simulink model "bitwise_calc"  (R2021a)
settings: Solver=FixedStepDiscrete  StartTime=0.0  StopTime=10.0  RelTol=1e-3  EnableMultiTasking=on
libraries: simulink x8
settings Model: Creator=Rana  LastModifiedBy=Rana
settings DataIOCC: ReturnWorkspaceOutputs=off
settings OptimizationCC: DefaultParameterBehavior=Inlined  InlineInvariantSignals=on  EnableMemcpy=off  LifeSpan=1  EfficientTunableParamExpr=on
settings DebuggingCC: UnderspecifiedInitializationDetection=Classic  MergeDetectMultiDrivingBlocksExec=none  SFMachineParentedDataDiag=warning  ArithmeticOperatorsInVariantConditions=warning
settings ModelReferenceCC: PropagateSignalLabelsOutOfModel=off
settings SFSimCC: MATLABDynamicMemAlloc=off  CustomCodeUndefinedFunction=UseInterfaceOnly
settings RTWCC: SystemTargetFile=ert.tlc  GenCodeOnly=on  TemplateMakefile=ert_default_tmf  GenerateReport=on  IncludeHyperlinkInReport=on  LaunchReport=on  GenerateTraceInfo=on  GenerateTraceReport=on  GenerateTraceReportSl=on  GenerateTraceReportSf=on  GenerateTraceReportEml=on
settings CodeAppCC: ForceParamTrailComments=on  IgnoreCustomStorageClasses=off  OperatorAnnotations=on  SimulinkDataObjDesc=on  SFDataObjDesc=on  MATLABFcnDesc=on  InsertBlockDesc=on  StateflowObjectComments=on  MATLABSourceComments=on
settings ERTTargetCC: MultiwordLength=2048  GenerateSampleERTMain=on  InlinedParameterPlacement=NonHierarchical  ERTCustomFileTemplate=example_file_process.tlc

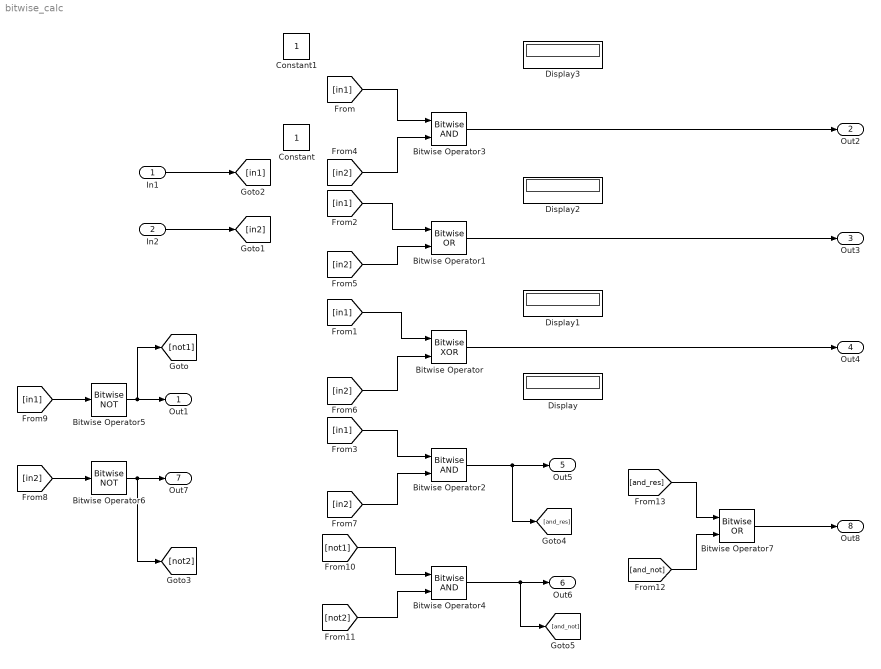
== system bitwise_calc ==
  In1 : Inport  OutDataTypeStr=uint8
  In2 : Inport  Port=2  OutDataTypeStr=uint8
  Bitwise Operator : simulink/Logic and Bit Operations/Bitwise Operator  logicop=XOR  UseBitMask=off  NumInputPorts=2  BitMask=bin2dec('11011001')  BitMaskRealWorld=Stored Integer
  Bitwise Operator1 : simulink/Logic and Bit Operations/Bitwise Operator  logicop=OR  UseBitMask=off  NumInputPorts=2  BitMask=bin2dec('11011001')  BitMaskRealWorld=Stored Integer
  Bitwise Operator2 : simulink/Logic and Bit Operations/Bitwise Operator  logicop=AND  UseBitMask=off  NumInputPorts=2  BitMask=bin2dec('11011001')  BitMaskRealWorld=Stored Integer
  Bitwise Operator3 : simulink/Logic and Bit Operations/Bitwise Operator  logicop=AND  UseBitMask=off  NumInputPorts=2  BitMask=bin2dec('11011001')  BitMaskRealWorld=Stored Integer
  Bitwise Operator4 : simulink/Logic and Bit Operations/Bitwise Operator  logicop=AND  UseBitMask=off  NumInputPorts=2  BitMask=bin2dec('11011001')  BitMaskRealWorld=Stored Integer
  Bitwise Operator5 : simulink/Logic and Bit Operations/Bitwise Operator  logicop=NOT  UseBitMask=off  BitMask=bin2dec('11011001')  BitMaskRealWorld=Stored Integer
  Bitwise Operator6 : simulink/Logic and Bit Operations/Bitwise Operator  logicop=NOT  UseBitMask=off  BitMask=bin2dec('11011001')  BitMaskRealWorld=Stored Integer
  Bitwise Operator7 : simulink/Logic and Bit Operations/Bitwise Operator  logicop=OR  UseBitMask=off  NumInputPorts=2  BitMask=bin2dec('11011001')  BitMaskRealWorld=Stored Integer
  Constant : Constant
  Constant1 : Constant
  Display{,1..3} (4 alike) : Display
  Out1 : Outport  SignalName=not1
  Out2 : Outport  Port=2  SignalName=and_res
  Out3 : Outport  Port=3  SignalName=or_res
  Out4 : Outport  Port=4  SignalName=xor_res
  Out5 : Outport  Port=5
  Out6 : Outport  Port=6
  Out7 : Outport  Port=7  SignalName=not2
  Out8 : Outport  Port=8  SignalName=xnor_res
  wires:
  In1/1 -> [in1]
  In2/1 -> [in2]
  [in1] -> Bitwise Operator3/1
  [in1] -> Bitwise Operator1/1
  [in1] -> Bitwise Operator/1
  [in1] -> Bitwise Operator2/1
  [in2] -> Bitwise Operator3/2
  [in2] -> Bitwise Operator1/2
  [in2] -> Bitwise Operator/2
  [in2] -> Bitwise Operator2/2
  Bitwise Operator3/1 -> Out2/1
  Bitwise Operator1/1 -> Out3/1
  Bitwise Operator/1 -> Out4/1
  Bitwise Operator2/1 -> [and_res], Out5/1
  [in1] -> Bitwise Operator5/1
  [in2] -> Bitwise Operator6/1
  Bitwise Operator5/1 -> [not1], Out1/1
  Bitwise Operator6/1 -> [not2], Out7/1
  Bitwise Operator4/1 -> [and_not], Out6/1
  Bitwise Operator7/1 -> Out8/1
  [not1] -> Bitwise Operator4/1
  [not2] -> Bitwise Operator4/2
  [and_res] -> Bitwise Operator7/1
  [and_not] -> Bitwise Operator7/2
